simulink model "FCS_MPC_6ph_Regelungsmodell"  (R2022a)
settings: Solver=ode23t  StartTime=0.0  StopTime=0.1  RelTol=1e-3  AbsTol=1e-3  EnableMultiTasking=on
values from neighbouring files (symbols this model uses):
  f_c = 100000    [Params_testbench.m]
  L_d = 0.0001473    [Params_testbench.m]
  L_q = 0.0001484    [Params_testbench.m]
  L_x = 0.00005566    (= 5.566e-05)    [Params_testbench.m]
  L_y = L_x    (= 5.566e-05)    [Params_testbench.m]
  p = 5    [Params_testbench.m]
  psi_pm = 0.0048    [Params_testbench.m]
  R_ph = 0.1278    [Params_testbench.m]
  T_100MHz = 1/f_100MHz    (= 1e-08)    [Params_testbench.m]
  u_dc = 36.0    (= 36)    [Params_testbench.m]
libraries: hdlsllib x53, nesl_utility x39, fl_lib x32, ee_lib x12, simulink x8, spsAlphaBetaZerotodq0Lib x1
(part 2 of 8)

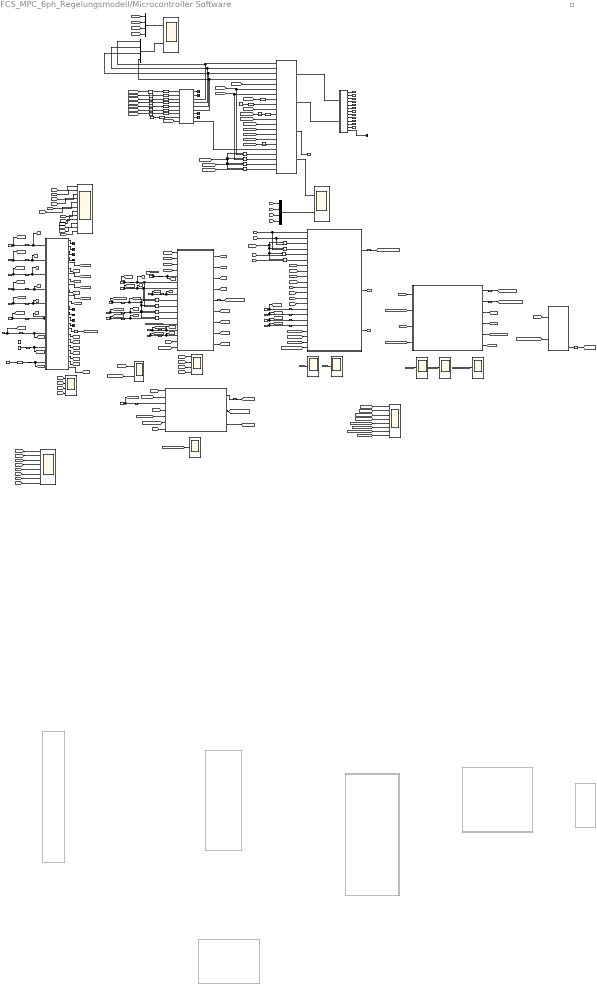
== system FCS_MPC_6ph_Regelungsmodell/Microcontroller Software ==
  note: IP-Core FCS_MPC_6Phase_PMSM
  note: IP-Core FCS_MPC_switching_states_2_level_inverter
  note: IP-Core VSD_and_Park_transformation
  i_a1 : Inport
  i_b1 : Inport  Port=2
  i_c1 : Inport  Port=3
  i_a2 : Inport  Port=4
  i_b2 : Inport  Port=5
  i_c2 : Inport  Port=6
  omega_m : Inport  Port=7
  theta_el : Inport  Port=8
  Rs : Inport  Port=9
  Ld : Inport  Port=10
  Lq : Inport  Port=11
  Lx : Inport  Port=12
  Ly : Inport  Port=13
  psiPM : Inport  Port=14
  SampleTime : Inport  Port=15
  id_ref : Inport  Port=16
  iq_ref : Inport  Port=17
  ix_ref : Inport  Port=18
  iy_ref : Inport  Port=19
  u_dc_link : Inport  Port=20
  pole_pairs : Inport  Port=21
  Ablauf : Scope  NumInputPorts=8
  Constant : Constant  Value=0
  Constant1 : Constant  Value=0  OutDataTypeStr=single  SampleTime=-1
  Constant2 : Constant  Value=0  OutDataTypeStr=fixdt(1,24,20)  SampleTime=-1
  Constant3 : Constant  Value=0
  Data Type Conversion{1..2,11..12} (4 alike) : DataTypeConversion  OutDataTypeStr=fixdt(1,24,20)  SaturateOnIntegerOverflow=off  RndMeth=Floor
  Data Type Conversion{5..10} (6 alike) : DataTypeConversion  OutDataTypeStr=fixdt(1,18,11)  SaturateOnIntegerOverflow=off  RndMeth=Floor
  Data Type Conversion13 : DataTypeConversion  OutDataTypeStr=fixdt(1,24,11)  SaturateOnIntegerOverflow=off  RndMeth=Floor
  Data Type Conversion4 : DataTypeConversion  OutDataTypeStr=boolean  RndMeth=Simplest  SaturateOnIntegerOverflow=off
  Delay1 : Delay  DelayLength=36
  Delay2 : Delay  DelayLength=21
  Delay22 : Delay  DelayLength=3
  Delay3 : Delay  DelayLength=66
  Delay4 : Delay  DelayLength=5
  Delay5 : Delay  DelayLength=5
  Delay6 : Delay
  Delay_compensation : Subsystem  TreatAsAtomicUnit=on
  Delay_compensation1 : Subsystem  Commented=on  TreatAsAtomicUnit=on
  Delay_compensation_phase_currents : Scope  NumInputPorts=4
  Divide{,1..11} (12 alike) : Product  Inputs=*/  RndMeth=Zero  SaturateOnIntegerOverflow=on
  Index : Scope
  J : Scope
  Min_cost_function_and_vopt1 : Subsystem  Commented=on  TreatAsAtomicUnit=on
  Min_cost_function_and_vopt2 : Subsystem  TreatAsAtomicUnit=on
  Mux : Mux
  Mux1 : Mux
  Mux2 : Mux
  Phase_voltages_per_switching_state1 : Subsystem  Commented=on  TreatAsAtomicUnit=on
  Phase_voltages_per_switching_state2 : Subsystem  TreatAsAtomicUnit=on
  Phase_voltages_per_switching_states : Scope
  Prediction_and_cost_function : Subsystem  TreatAsAtomicUnit=on
  Prediction_and_cost_function1 : Subsystem  Commented=on  TreatAsAtomicUnit=on
  Pulse Generator3 : DiscretePulseGenerator  PulseType=Time based  Period=1/100000  PulseWidth=0.1
  Pulse Generator4 : DiscretePulseGenerator  Commented=on  PulseType=Time based  Period=1/100000  PulseWidth=5
  Rate Transition{1..23} (23 alike) : RateTransition  OutPortSampleTime=1.0000e-08
  Subsystem2 : Subsystem
  Subsystem3 : Subsystem
  Subsystem5 : Subsystem  TreatAsAtomicUnit=on
  Switching_states : Subsystem  TreatAsAtomicUnit=on
  Switching_states1 : Subsystem  Commented=on  TreatAsAtomicUnit=on
  Terminator{,1..12} (13 alike) : Terminator
  Unit Delay{1..9} (9 alike) : UnitDelay  SampleTime=1/f_c  HasFrameUpgradeWarning=on
  VSD_and_Park_transformed_phase_currents : Scope  NumInputPorts=4
  last_applied_optimal_voltages : Scope
  min_Index_AXI : Scope
  min_J_AXI : Scope
  phase_currents : Scope  NumInputPorts=8
  phase_currents1 : Scope  NumInputPorts=12
  phase_currents2 : Scope  NumInputPorts=2
  phase_currents3 : Scope  NumInputPorts=2
  theta_test : Scope  NumInputPorts=2
  vsd_and_park_tra : Subsystem  TreatAsAtomicUnit=on
  vsd_and_park_tra1 : Subsystem  Commented=on  TreatAsAtomicUnit=on
  HB1T1 : Outport
  HB1B1 : Outport  Port=2
  HB2T1 : Outport  Port=3
  HB2B1 : Outport  Port=4
  HB3T1 : Outport  Port=5
  HB3B1 : Outport  Port=6
  HB4T : Outport  Port=7
  HB4B : Outport  Port=8
  HB5T : Outport  Port=9
  HB5B : Outport  Port=10
  HB6T : Outport  Port=11
  HB6B : Outport  Port=12
  v_opt : Outport  Port=13
  wires:
  Pulse Generator3/1 -> Data Type Conversion4/1
  vsd_and_park_tra/17(done) -> Delay22/1
  vsd_and_park_tra/4(i_beta_axi) -> Terminator1/1
  vsd_and_park_tra/10(i_x_axi) -> [i_x_AXI]
  vsd_and_park_tra/16(i_0_minus_axi) -> Terminator7/1
  Constant1/1 -> Rate Transition7/1  "i_a1_IP_Core"
  vsd_and_park_tra/12(i_y_axi) -> [i_y_AXI]
  vsd_and_park_tra/14(i_0_plus_axi) -> Terminator6/1
  vsd_and_park_tra/8(i_q_axi) -> [i_q_AXI]
  vsd_and_park_tra/6(i_d_axi) -> [i_d_AXI]
  vsd_and_park_tra/2(i_alpha_axi) -> Terminator/1
  i_a1/1 -> Rate Transition23/1, [i_a1_without_RT]  "i_a1_IP_Core"
  i_c2/1 -> Rate Transition5/1, [i_c2_without_RT]  "i_c2_IP_Core"
  i_b2/1 -> Rate Transition4/1, [i_b2_without_RT]  "i_b2_IP_Core"
  i_a2/1 -> Rate Transition3/1, [i_a2_without_RT]  "i_a2_IP_Core"
  i_c1/1 -> Rate Transition2/1, [i_c1_without_RT]  "i_c1_IP_Core"
  i_b1/1 -> Rate Transition1/1, [i_b1_without_RT]  "i_b1_IP_Core"
  vsd_and_park_tra/1(i_alpha) -> Terminator9/1  "i_alpha"
  vsd_and_park_tra/3(i_beta) -> Terminator10/1  "i_beta"
  vsd_and_park_tra/13(i_0_plus) -> Terminator11/1  "i_0_plus"
  vsd_and_park_tra/15(i_0_minus) -> Terminator12/1  "i_0_minus"
  vsd_and_park_tra/18(i_a1_axi) -> [i_a1_AXI]
  vsd_and_park_tra/19(i_b1_axi) -> [i_b1_AXI]
  vsd_and_park_tra/20(i_c1_axi) -> [i_c1_AXI]
  vsd_and_park_tra/21(i_a2_axi) -> [i_a2_AXI]
  vsd_and_park_tra/22(i_b2_axi) -> [i_b2_AXI]
  vsd_and_park_tra/23(i_c2_axi) -> [i_c2_AXI]
  [i_a1_AXI] -> phase_currents1/1
  [i_b1_AXI] -> phase_currents1/2
  [i_c1_AXI] -> phase_currents1/3
  [i_a2_AXI] -> phase_currents1/4
  [i_b2_AXI] -> phase_currents1/5
  [i_c2_AXI] -> phase_currents1/6
  [i_d_AXI] -> VSD_and_Park_transformed_phase_currents/1
  [i_q_AXI] -> VSD_and_Park_transformed_phase_currents/2
  [i_y_AXI] -> VSD_and_Park_transformed_phase_currents/4
  [i_x_AXI] -> VSD_and_Park_transformed_phase_currents/3
  Divide1/1 -> Delay_compensation/10(SampleTime_div_Lq_AXI)
  Divide/1 -> Delay_compensation/9(SampleTime_div_Ld_AXI)
  Delay_compensation/2(iq_k_1) -> [iq_k_1]
  Divide2/1 -> Delay_compensation/11(SampleTime_div_Lx_AXI)
  Delay_compensation/1(id_k_1) -> [id_k_1]
  Delay_compensation/4(iy_k_1) -> [iy_k_1]
  Delay_compensation/3(ix_k_1) -> [ix_k_1]
  Divide3/1 -> Delay_compensation/12(SampleTime_div_Ly_AXI)
  psiPM/1 -> Rate Transition9/1, [psiPM_without_RT]  "i_d"
  Lq/1 -> Rate Transition10/1, [Lq_without_RT]  "i_a1_IP_Core"
  Ld/1 -> Rate Transition11/1, [Ld_without_RT]  "i_a1_IP_Core"
  Rs/1 -> Rate Transition12/1, [Rs_without_RT]  "i_a1_IP_Core"
  Lx/1 -> Rate Transition14/1, [Lx_without_RT]  "i_a1_IP_Core"
  Ly/1 -> Rate Transition15/1, [Ly_without_RT]  "i_a1_IP_Core"
  pole_pairs/1 -> Rate Transition16/1, [pole_pairs_without_RT]  "i_a1_IP_Core"
  omega_m/1 -> Rate Transition17/1, [omega_m_without_RT]  "i_d"
  [valid_in_ADC] -> Delay_compensation/16(valid_in_ADC)
  [done_VSD_and_Park] -> Delay_compensation/17(valid_in)
  vsd_and_park_tra/5(i_d) -> [i_d_measured]  "i_d"
  vsd_and_park_tra/7(i_q) -> [i_q_measured]  "i_q"
  vsd_and_park_tra/9(i_x) -> [i_x_measured]  "i_x"
  vsd_and_park_tra/11(i_y) -> [i_y_measured]  "i_y"
  [i_d_measured] -> Delay_compensation/1(id_measured)
  [i_q_measured] -> Delay_compensation/2(iq_measured)
  [i_x_measured] -> Delay_compensation/3(ix_measured)
  [i_y_measured] -> Delay_compensation/4(iy_measured)
  Delay_compensation/6(id_k_1_AXI) -> [id_k_1_AXI]
  Delay_compensation/7(iq_k_1_AXI) -> [iq_k_1_AXI]
  Delay_compensation/8(ix_k_1_AXI) -> [ix_k_1_AXI]
  Delay_compensation/9(iy_k_1_AXI) -> [iy_k_1_AXI]
  [id_k_1_AXI] -> Delay_compensation_phase_currents/1
  [iq_k_1_AXI] -> Delay_compensation_phase_currents/2
  [ix_k_1_AXI] -> Delay_compensation_phase_currents/3
  [iy_k_1_AXI] -> Delay_compensation_phase_currents/4
  [theta_el] -> Phase_voltages_per_switching_state2/1(theta_el)
  [theta_el_offset_AXI] -> Phase_voltages_per_switching_state2/2(theta_el_offset_AXI)
  u_dc_link/1 -> Rate Transition22/1, [u_dc_link_without_RT]  "i_a1_IP_Core"
  Delay_compensation/5(done) -> Delay1/1
  [valid_in_delay_compensation] -> Phase_voltages_per_switching_state2/5(valid_in_delay_compensation)
  [valid_in_ADC] -> Phase_voltages_per_switching_state2/7(valid_in_ADC)
  Phase_voltages_per_switching_state2/1(done) -> Delay2/1
  Phase_voltages_per_switching_state2/2(phase_voltages_per_switching_state) -> [phase_voltages_per_switching_states]
  [phase_voltages_per_switching_states] -> Phase_voltages_per_switching_states/1
  Divide6/1 -> Prediction_and_cost_function/5(SampleTime_div_Lx_AXI)
  [psiPM] -> Prediction_and_cost_function/14(psiPM_AXI)
  Divide7/1 -> Prediction_and_cost_function/6(SampleTime_div_Ly_AXI)
  [Ld] -> Divide4/2, Prediction_and_cost_function/2(Ld_AXI)
  [omega_m] -> Prediction_and_cost_function/12(omega_m_measured)
  [SampleTime] -> Divide5/1, Divide7/1, Divide6/1, Divide4/1
  [Lq] -> Divide5/2, Prediction_and_cost_function/1(Lq_AXI)
  Divide4/1 -> Prediction_and_cost_function/3(SampleTime_div_Ld_AXI)
  [Rs] -> Prediction_and_cost_function/11(Rs_AXI)
  [Ly] -> Divide7/2
  [Lx] -> Divide6/2
  Prediction_and_cost_function/2(Index) -> [Index]
  Divide5/1 -> Prediction_and_cost_function/4(SampleTime_div_Lq_AXI)
  [pole_pairs] -> Prediction_and_cost_function/13(pole_pairs_AXI)
  Prediction_and_cost_function/3(J) -> [J]
  [J] -> J/1
  [Index] -> Index/1
  Prediction_and_cost_function/1(done) -> Delay3/1
  [id_k_1] -> Prediction_and_cost_function/7(id_k_1)
  [iq_k_1] -> Prediction_and_cost_function/8(iq_k_1)
  [ix_k_1] -> Prediction_and_cost_function/9(ix_k_1)
  [iy_k_1] -> Prediction_and_cost_function/10(iy_k_1)
  id_ref/1 -> Rate Transition18/1, [id_ref_without_RT]  "i_a1_IP_Core"
  iq_ref/1 -> Rate Transition19/1, [iq_ref_without_RT]  "i_a1_IP_Core"
  ix_ref/1 -> Rate Transition20/1, [ix_ref_without_RT]  "i_a1_IP_Core"
  iy_ref/1 -> Rate Transition21/1, [iy_ref_without_RT]  "i_a1_IP_Core"
  [valid_in_phase_voltages] -> Prediction_and_cost_function/19(valid_in)
  [done_VSD_and_Park] -> Prediction_and_cost_function/20(Reset)
  [valid_in_ADC] -> Prediction_and_cost_function/21(valid_in_ADC)
  [phase_voltages_per_switching_states] -> Prediction_and_cost_function/22(dqxy_phase_voltage_per_switching_state)
  Min_cost_function_and_vopt2/6(Index_AXI) -> [min_Index_AXI]
  Min_cost_function_and_vopt2/2(done_complete) -> Delay5/1
  Min_cost_function_and_vopt2/3(J_AXI) -> [min_J_AXI]
  Min_cost_function_and_vopt2/1(done) -> Delay4/1
  Min_cost_function_and_vopt2/4(Index) -> [min_Index]
  Min_cost_function_and_vopt2/5(voltages) -> [last_applied_optimal_voltages]
  [Index] -> Min_cost_function_and_vopt2/1(Index_in)
  [Index] -> Phase_voltages_per_switching_state2/4(Index)
  [valid_in_prediction_and_cost_function] -> Min_cost_function_and_vopt2/2(valid_in)
  [J] -> Min_cost_function_and_vopt2/3(J_in)
  [phase_voltages_per_switching_states] -> Min_cost_function_and_vopt2/4(phase_voltages_per_switching_state_in)
  [min_J_AXI] -> min_J_AXI/1
  [min_Index_AXI] -> min_Index_AXI/1
  [last_applied_optimal_voltages] -> last_applied_optimal_voltages/1
  [last_applied_optimal_voltages] -> Delay_compensation/13(last_applied_optimal_voltages_in)
  [valid_in_done_min_cost_function] -> Phase_voltages_per_switching_state2/6(valid_in_min_cost_function-and_vopt)
  Switching_states/13(done) -> Delay6/1
  [min_Index] -> Switching_states/1(I)
  [valid_in_done_complete_min_cost_function] -> Switching_states/2(valid_in)
  [valid_in_ADC] -> Ablauf/1  "valid_in_ADC"
  [done_VSD_and_Park] -> Ablauf/2  "done_VSD_and_Park"
  [valid_in_delay_compensation] -> Ablauf/3  "done_delay_compensation"
  [valid_in_phase_voltages] -> Ablauf/4  "done_phase_voltages"
  [valid_in_prediction_and_cost_function] -> Ablauf/5  "done_prediction_and_cost_function"
  [valid_in_done_min_cost_function] -> Ablauf/6  "done_min_cost_function"
  [valid_in_done_complete_min_cost_function] -> Ablauf/7  "done_complete_min_cost_function"
  [done_switching_states] -> Ablauf/8  "done_switching_states"
  Delay22/1 -> [done_VSD_and_Park]
  Delay1/1 -> [valid_in_delay_compensation]
  Delay2/1 -> [valid_in_phase_voltages]
  Delay3/1 -> [valid_in_prediction_and_cost_function]
  Delay4/1 -> [valid_in_done_min_cost_function]
  Delay5/1 -> [valid_in_done_complete_min_cost_function]
  Delay6/1 -> [done_switching_states]
  [id_k_1_AXI] -> phase_currents/1  "id_k_1"
  [iq_k_1_AXI] -> phase_currents/2  "iq_k_1"
  [ix_k_1_AXI] -> phase_currents/3  "ix_k_1"
  [iy_k_1_AXI] -> phase_currents/4  "iy_k_1"
  [i_d_AXI] -> phase_currents/5  "id"
  [i_q_AXI] -> phase_currents/6  "iq"
  [i_x_AXI] -> phase_currents/7  "ix"
  [i_y_AXI] -> phase_currents/8  "iy"
  Data Type Conversion4/1 -> Rate Transition8/1  "i_a1_IP_Core"
  SampleTime/1 -> Rate Transition13/1, [SampleTime_without_RT]  "i_a1_IP_Core"
  [i_a1] -> phase_currents1/7
  [i_b1] -> phase_currents1/8
  [i_c1] -> phase_currents1/9
  [i_a2] -> phase_currents1/10
  [i_b2] -> phase_currents1/11
  [i_c2] -> phase_currents1/12
  vsd_and_park_tra/24(theta_test) -> [theta_test_vsd]
  [theta_test_vsd] -> theta_test/1  "VSD"
  Phase_voltages_per_switching_state2/3(theta_test) -> [theta_test_phase_voltages]
  [theta_test_phase_voltages] -> theta_test/2  "phase_voltages"
  theta_el/1 -> Rate Transition6/1, [theta_el_without_RT]  "i_a1_IP_Core"
  Constant/1 -> Data Type Conversion1/1
  Divide11/1 -> Subsystem3/22(SampleTime_div_Ly_AXI)  "i_d"
  Subsystem2/1(i_alpha) -> Terminator4/1  "i_alpha"
  Subsystem3/1(I) -> Subsystem5/1(I)
  [Ld_without_RT] -> Subsystem3/6(Ld_AXI), Divide8/2  "i_d"
  Divide8/1 -> Subsystem3/19(SampleTime_div_Ld_AXI)  "i_d"
  Subsystem2/6(i_y) -> Subsystem3/4(i_y), Mux1/4  "i_y"
  Data Type Conversion2/1 -> Subsystem3/9(theta_el_offset_AXI)  "curent_valid_in"
  Divide10/1 -> Subsystem3/21(SampleTime_div_Lx_AXI)  "i_d"
  Constant3/1 -> Data Type Conversion2/1
  Subsystem2/5(i_x) -> Subsystem3/3(i_x), Mux1/3  "i_x"
  Subsystem3/3(v_opt) -> v_opt/1
  [Rs_without_RT] -> Subsystem3/5(Rs_AXI)  "i_d"
  Subsystem5/13(done) -> Terminator8/1  "done_switching_states"
  [Lq_without_RT] -> Divide9/2, Subsystem3/7(Lq_AXI)  "i_d"
  Subsystem2/4(i_q) -> Mux1/2, Subsystem3/2(i_q)  "i_q"
  Subsystem3/2(done) -> Subsystem5/2(valid_in)  "done_MPC"
  Subsystem2/3(i_d) -> Mux1/1, Subsystem3/1(i_d)  "i_d"
  Subsystem2/9(done) -> Subsystem3/18(valid_in)  "done_trans"
  [Ly_without_RT] -> Divide11/2
  [SampleTime_without_RT] -> Divide8/1, Divide9/1, Divide11/1, Divide10/1
  Divide9/1 -> Subsystem3/20(SampleTime_div_Lq_AXI)  "i_d"
  Subsystem2/2(i_beta) -> Terminator5/1  "i_beta"
  [Lx_without_RT] -> Divide10/2
  Subsystem2/8(i_0_minus) -> Terminator3/1  "i_0_minus"
  Data Type Conversion1/1 -> Subsystem2/8(theta_el_offset_AXI)  "curent_valid_in"
  Subsystem2/7(i_0_plus) -> Terminator2/1  "i_0_plus"
  Data Type Conversion5/1 -> Subsystem2/1(i_a1)  "curent_valid_in"
  Data Type Conversion6/1 -> Subsystem2/2(i_b1)  "curent_valid_in"
  Data Type Conversion7/1 -> Subsystem2/3(i_c1)  "curent_valid_in"
  Data Type Conversion8/1 -> Subsystem2/4(i_a2)  "curent_valid_in"
  Data Type Conversion9/1 -> Subsystem2/5(i_b2)  "curent_valid_in"
  Data Type Conversion10/1 -> Subsystem2/6(i_c2)  "curent_valid_in"
  [theta_el_without_RT] -> Unit Delay7/1  "curent_valid_in"
  [theta_el_without_RT] -> Data Type Conversion12/1
  Data Type Conversion11/1 -> Subsystem2/7(theta_el)  "curent_valid_in"
  Data Type Conversion12/1 -> Subsystem3/8(theta_el)  "curent_valid_in"
  [psiPM_without_RT] -> Subsystem3/10(psiPM_AXI)
  [pole_pairs_without_RT] -> Subsystem3/12(pole_pairs_AXI)
  [id_ref_without_RT] -> Subsystem3/13(id_ref_AXI)
  [iq_ref_without_RT] -> Subsystem3/14(iq_ref_AXI)
  [ix_ref_without_RT] -> Subsystem3/15(ix_ref_AXI)
  [iy_ref_without_RT] -> Subsystem3/16(iy_ref_AXI)
  Data Type Conversion13/1 -> Subsystem3/11(omega_m)
  [valid_in_ADC] -> Subsystem2/9(curent_valid_in)  "curent_valid_in"
  Mux/1 -> phase_currents2/1
  [i_d_measured] -> Mux/1
  [i_q_measured] -> Mux/2
  [i_x_measured] -> Mux/3
  [i_y_measured] -> Mux/4
  Mux1/1 -> phase_currents2/2
  [i_a1_without_RT] -> Unit Delay2/1
  [i_b1_without_RT] -> Unit Delay1/1
  [i_c1_without_RT] -> Unit Delay3/1
  [i_a2_without_RT] -> Unit Delay4/1
  [i_b2_without_RT] -> Unit Delay5/1
  [i_c2_without_RT] -> Unit Delay6/1
  [omega_m_without_RT] -> Unit Delay8/1
  [u_dc_link_without_RT] -> Unit Delay9/1
  Rate Transition23/1 -> [i_a1], vsd_and_park_tra/1(i_a1)  "i_a1_IP_Core"
  Rate Transition1/1 -> [i_b1], vsd_and_park_tra/2(i_b1)  "i_a1_IP_Core"
  Rate Transition2/1 -> [i_c1], vsd_and_park_tra/3(i_c1)  "i_a1_IP_Core"
  Rate Transition3/1 -> [i_a2], vsd_and_park_tra/4(i_a2)  "i_a1_IP_Core"
  Rate Transition4/1 -> [i_b2], vsd_and_park_tra/5(i_b2)  "i_a1_IP_Core"
  Rate Transition5/1 -> [i_c2], vsd_and_park_tra/6(i_c2)  "i_a1_IP_Core"
  Rate Transition6/1 -> [theta_el], vsd_and_park_tra/7(theta_el)  "i_a1_IP_Core"
  Rate Transition7/1 -> vsd_and_park_tra/8(theta_el_offset_), [theta_el_offset_AXI]  "i_a1_IP_Core"
  Rate Transition8/1 -> [valid_in_ADC], vsd_and_park_tra/9(curent_valid_in)  "i_a1_IP_Core"
  Rate Transition9/1 -> [psiPM], Delay_compensation/5(psiPM_AXI)  "i_a1_IP_Core"
  Rate Transition10/1 -> [Lq], Delay_compensation/6(Lq_AXI), Divide1/2  "i_a1_IP_Core"
  Rate Transition11/1 -> [Ld], Delay_compensation/7(Ld_AXI), Divide/2  "i_a1_IP_Core"
  Rate Transition12/1 -> [Rs], Delay_compensation/8(Rs_AXI)  "i_a1_IP_Core"
  Rate Transition13/1 -> Divide/1, Divide1/1, Divide3/1, Divide2/1, [SampleTime]  "i_a1_IP_Core"
  Rate Transition14/1 -> [Lx], Divide2/2  "i_a1_IP_Core"
  Rate Transition15/1 -> [Ly], Divide3/2  "i_a1_IP_Core"
  Rate Transition16/1 -> [pole_pairs], Delay_compensation/14(pole_pairs_AXI)  "i_a1_IP_Core"
  Rate Transition17/1 -> [omega_m], Delay_compensation/15(omega_m_measured)  "i_a1_IP_Core"
  Rate Transition18/1 -> Prediction_and_cost_function/15(id_ref_AXI)  "i_a1_IP_Core"
  Rate Transition19/1 -> Prediction_and_cost_function/16(iq_ref_AXI)  "i_a1_IP_Core"
  Rate Transition20/1 -> Prediction_and_cost_function/17(ix_ref_AXI)  "i_a1_IP_Core"
  Rate Transition21/1 -> Prediction_and_cost_function/18(iy_ref_AXI)  "i_a1_IP_Core"
  Rate Transition22/1 -> Phase_voltages_per_switching_state2/3(u_dc_link_voltage_AXI)  "i_a1_IP_Core"
  Unit Delay2/1 -> Data Type Conversion5/1
  Unit Delay1/1 -> Data Type Conversion6/1
  Unit Delay3/1 -> Data Type Conversion7/1
  Unit Delay4/1 -> Data Type Conversion8/1
  Unit Delay5/1 -> Data Type Conversion9/1
  Unit Delay6/1 -> Data Type Conversion10/1
  Unit Delay7/1 -> Data Type Conversion11/1
  Unit Delay8/1 -> Data Type Conversion13/1
  Unit Delay9/1 -> Subsystem3/17(u_dc_link_AXI)
  Subsystem5/2(HB1B) -> HB1B1/1
  Subsystem5/1(HB1T) -> HB1T1/1
  Subsystem5/3(HB2T) -> HB2T1/1
  Subsystem5/4(HB2B) -> HB2B1/1
  Subsystem5/5(HB3T) -> HB3T1/1
  Subsystem5/6(HB3B) -> HB3B1/1
  Subsystem5/7(HB4T) -> HB4T/1
  Subsystem5/8(HB4B) -> HB4B/1
  Subsystem5/9(HB5T) -> HB5T/1
  Subsystem5/10(HB5B) -> HB5B/1
  Subsystem5/11(HB6T) -> HB6T/1
  Subsystem5/12(HB6B) -> HB6B/1
  Subsystem3/4(Prediction_old) -> phase_currents3/1
  [id_k_1] -> Mux2/1
  [iq_k_1] -> Mux2/2
  [ix_k_1] -> Mux2/3
  [iy_k_1] -> Mux2/4
  Mux2/1 -> phase_currents3/2

== system FCS_MPC_6ph_Regelungsmodell/Power_Source ==
  Controlled Voltage Source : fl_lib/Electrical/Electrical Sources/Controlled Voltage Source
      settings: SourceProductBaseCode=PW,SS,VE
  + : PMIOPort  Side=Right
  - : PMIOPort  Port=2  Side=Right
  ref_voltage : PMIOPort  Port=3  Side=Left
  connections:
  Controlled Voltage Source/LConn1 -- +/RConn1
  Controlled Voltage Source/RConn2 -- -/RConn1
  Controlled Voltage Source/RConn1 -- ref_voltage/RConn1

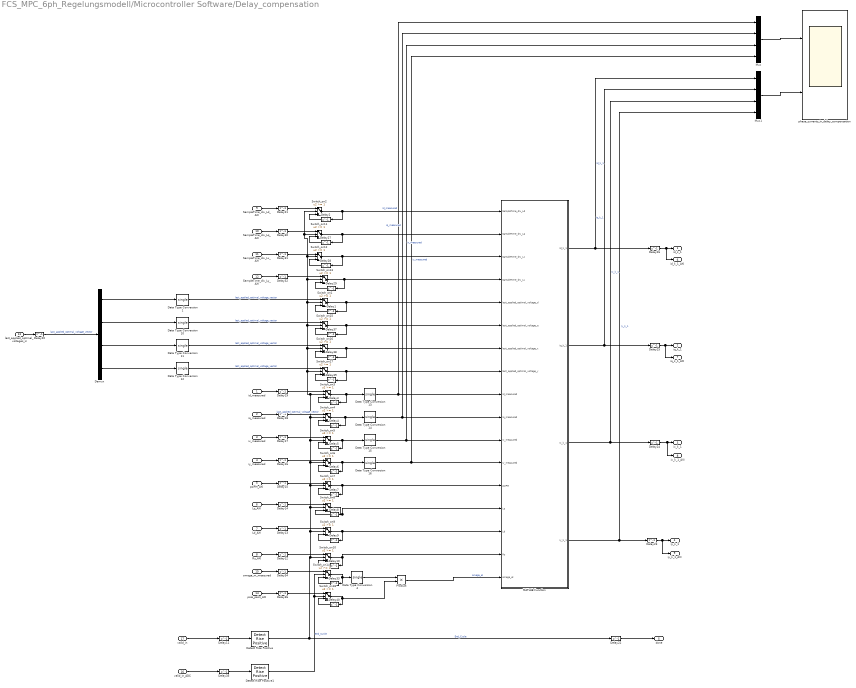
== system FCS_MPC_6ph_Regelungsmodell/Microcontroller Software/Delay_compensation ==
  id_measured : Inport
  iq_measured : Inport  Port=2
  ix_measured : Inport  Port=3
  iy_measured : Inport  Port=4
  psiPM_AXI : Inport  Port=5
  Lq_AXI : Inport  Port=6
  Ld_AXI : Inport  Port=7
  Rs_AXI : Inport  Port=8
  SampleTime_div_Ld_AXI : Inport  Port=9
  SampleTime_div_Lq_AXI : Inport  Port=10
  SampleTime_div_Lx_AXI : Inport  Port=11
  SampleTime_div_Ly_AXI : Inport  Port=12
  last_applied_optimal_voltages_in : Inport  Port=13
  pole_pairs_AXI : Inport  Port=14
  omega_m_measured : Inport  Port=15
  valid_in_ADC : Inport  Port=16
  valid_in : Inport  Port=17
  Data Type Conversion{1,4,10..16} (9 alike) : DataTypeConversion  OutDataTypeStr=single  RndMeth=Nearest  SaturateOnIntegerOverflow=off
  Delay{1..40} (40 alike) : Delay  DelayLength=1
  Demux : Demux
  Detect Rise Positive : hdlsllib/Logic and Bit Operations/Detect Rise Positive  vinit=0  OutDataTypeStr=boolean
      settings: SourceProductBaseCode=SL
  Detect Rise Positive1 : hdlsllib/Logic and Bit Operations/Detect Rise Positive  vinit=0  OutDataTypeStr=boolean
      settings: SourceProductBaseCode=SL
  MATLAB Function : MATLAB Function  TreatAsAtomicUnit=on
  Mux : Mux
  Mux1 : Mux
  Product : Product  Inputs=**
  Switch_on{1..13,15..18} (17 alike) : Switch  Threshold=1  OutDataTypeStr=single  RndMeth=Simplest  SaturateOnIntegerOverflow=off  InputSameDT=off
  Switch_on14 : Switch  Threshold=1  RndMeth=Simplest  SaturateOnIntegerOverflow=off  InputSameDT=off  OutDataTypeStr=Inherit: Same as first input
  phase_currents_in_delay_compensation : Scope  NumInputPorts=2
  id_k_1 : Outport
  iq_k_1 : Outport  Port=2
  ix_k_1 : Outport  Port=3
  iy_k_1 : Outport  Port=4
  done : Outport  Port=5
  id_k_1_AXI : Outport  Port=6
  iq_k_1_AXI : Outport  Port=7
  ix_k_1_AXI : Outport  Port=8
  iy_k_1_AXI : Outport  Port=9
  wires:
  Switch_on14/1 -> Data Type Conversion4/1, Delay33/1
  Delay33/1 -> Switch_on14/3
  pole_pairs_AXI/1 -> Delay36/1
  Delay9/1 -> Switch_on9/3
  Switch_on9/1 -> Delay9/1, MATLAB Function/15(Ld)
  Delay32/1 -> Switch_on13/1
  Lq_AXI/1 -> Delay14/1
  Delay31/1 -> Switch_on12/1
  Switch_on12/1 -> Delay28/1, MATLAB Function/3(SampleTime_div_Lx)
  Delay30/1 -> Switch_on11/1
  Delay29/1 -> Switch_on13/3
  SampleTime_div_Lx_AXI/1 -> Delay31/1
  Delay26/1 -> id_k_1_AXI/1, id_k_1/1
  Product/1 -> MATLAB Function/17(omega_el)  "omega_el"
  Delay11/1 -> Detect Rise Positive/1
  Delay2/1 -> Switch_on2/3
  SampleTime_div_Lq_AXI/1 -> Delay30/1
  Switch_on5/1 -> Delay5/1, Data Type Conversion15/1
  Delay12/1 -> Switch_on10/1
  Rs_AXI/1 -> Delay12/1
  Delay1/1 -> Switch_on1/3
  Delay27/1 -> Switch_on11/3
  Delay21/1 -> Switch_on2/1
  Delay23/1 -> iy_k_1_AXI/1, iy_k_1/1
  Delay24/1 -> ix_k_1_AXI/1, ix_k_1/1
  Delay20/1 -> Demux/1  "last_applied_optimal_voltage_vector"
  Switch_on1/1 -> Delay1/1, MATLAB Function/5(last_applied_optimal_voltage_d)
  Delay8/1 -> Switch_on8/3
  Delay10/1 -> Switch_on10/3
  valid_in/1 -> Delay11/1
  Switch_on6/1 -> Delay6/1, Data Type Conversion16/1
  psiPM_AXI/1 -> Delay15/1
  Delay25/1 -> iq_k_1_AXI/1, iq_k_1/1
  Switch_on13/1 -> Delay29/1, MATLAB Function/4(SampleTime_div_Ly)
  Switch_on4/1 -> Delay4/1, Data Type Conversion14/1
  Delay15/1 -> Switch_on7/1
  SampleTime_div_Ly_AXI/1 -> Delay32/1
  Switch_on10/1 -> Delay10/1, MATLAB Function/16(Rs)
  Delay7/1 -> Switch_on7/3
  Delay28/1 -> Switch_on12/3
  Switch_on8/1 -> Delay8/1, MATLAB Function/14(Lq)
  Ld_AXI/1 -> Delay13/1
  Delay6/1 -> Switch_on6/3
  Delay4/1 -> Switch_on4/3
  Switch_on11/1 -> Delay27/1, MATLAB Function/2(SampleTime_div_Lq)
  Delay3/1 -> Switch_on3/3
  Delay14/1 -> Switch_on8/1
  Switch_on2/1 -> Delay2/1, MATLAB Function/1(SampleTime_div_Ld)
  Delay22/1 -> done/1
  Switch_on3/1 -> Delay3/1, Data Type Conversion13/1
  Delay13/1 -> Switch_on9/1
  Delay5/1 -> Switch_on5/3
  SampleTime_div_Ld_AXI/1 -> Delay21/1
  last_applied_optimal_voltages_in/1 -> Delay20/1
  id_measured/1 -> Delay19/1
  iq_measured/1 -> Delay18/1
  ix_measured/1 -> Delay17/1
  iy_measured/1 -> Delay16/1
  omega_m_measured/1 -> Delay34/1
  Delay35/1 -> Detect Rise Positive1/1
  valid_in_ADC/1 -> Delay35/1
  Delay34/1 -> Switch_on14/1
  Delay36/1 -> Switch_on18/1
  Demux/1 -> Data Type Conversion1/1
  Delay37/1 -> Switch_on15/3
  Switch_on15/1 -> MATLAB Function/6(last_applied_optimal_voltage_q), Delay37/1
  Demux/2 -> Data Type Conversion10/1
  Delay38/1 -> Switch_on16/3
  Switch_on16/1 -> MATLAB Function/7(last_applied_optimal_voltage_x), Delay38/1
  Demux/3 -> Data Type Conversion11/1
  Delay39/1 -> Switch_on17/3
  Detect Rise Positive/1 -> Switch_on17/2, Switch_on16/2, Switch_on15/2, Switch_on13/2, Switch_on2/2, Switch_on11/2, Switch_on12/2, Switch_on1/2, Switch_on3/2, Switch_on4/2, Switch_on5/2, Switch_on6/2, Switch_on7/2, Switch_on8/2, Switch_on9/2, Switch_on10/2, Delay22/1  "End_Cycle"
  Switch_on17/1 -> MATLAB Function/8(last_applied_optimal_voltage_y), Delay39/1
  Demux/4 -> Data Type Conversion12/1
  Data Type Conversion1/1 -> Switch_on1/1  "last_applied_optimal_voltage_vector"
  Data Type Conversion10/1 -> Switch_on15/1  "last_applied_optimal_voltage_vector"
  Data Type Conversion11/1 -> Switch_on16/1  "last_applied_optimal_voltage_vector"
  Data Type Conversion12/1 -> Switch_on17/1  "last_applied_optimal_voltage_vector"
  Delay19/1 -> Switch_on3/1
  Delay18/1 -> Switch_on4/1  "last_applied_optimal_voltage_vector"
  Delay17/1 -> Switch_on5/1
  Delay16/1 -> Switch_on6/1
  Data Type Conversion4/1 -> Product/1
  MATLAB Function/1(id_k_1) -> Mux1/1, Delay26/1  "id_k_1"
  MATLAB Function/2(iq_k_1) -> Mux1/2, Delay25/1  "iq_k_1"
  MATLAB Function/3(ix_k_1) -> Mux1/3, Delay24/1  "ix_k_1"
  MATLAB Function/4(iy_k_1) -> Mux1/4, Delay23/1  "iy_k_1"
  Switch_on18/1 -> Product/2, Delay40/1
  Detect Rise Positive1/1 -> Switch_on18/2, Switch_on14/2  "End_Cycle"
  Delay40/1 -> Switch_on18/3
  Data Type Conversion13/1 -> Mux/1, MATLAB Function/9(id_measured)  "id_measured"
  Data Type Conversion14/1 -> Mux/2, MATLAB Function/10(iq_measured)  "iq_measured"
  Data Type Conversion15/1 -> Mux/3, MATLAB Function/11(ix_measured)  "ix_measured"
  Data Type Conversion16/1 -> Mux/4, MATLAB Function/12(iy_measured)  "iy_measured"
  Switch_on7/1 -> MATLAB Function/13(psiPM), Delay7/1
  Mux/1 -> phase_currents_in_delay_compensation/1
  Mux1/1 -> phase_currents_in_delay_compensation/2

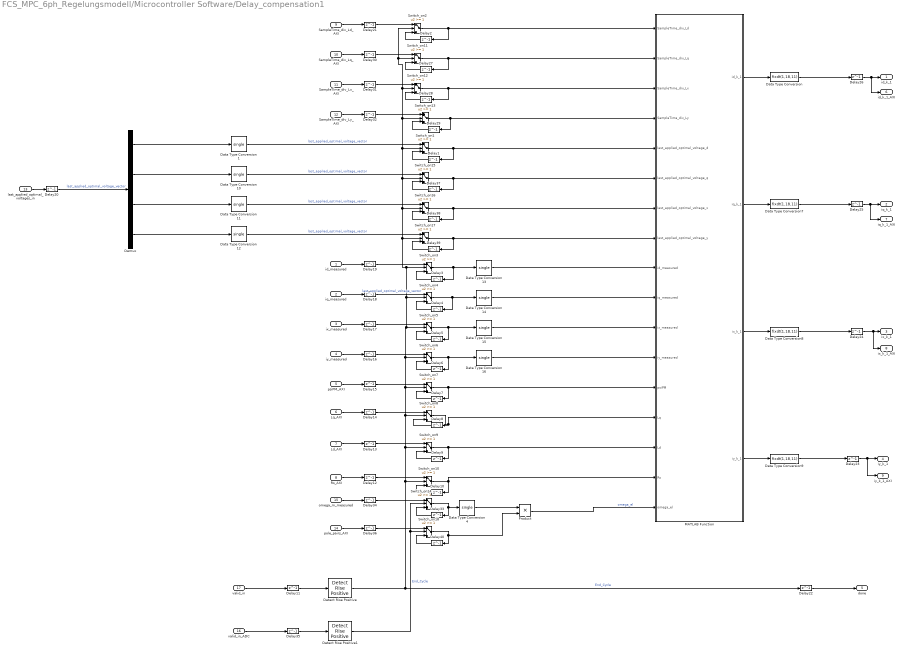
== system FCS_MPC_6ph_Regelungsmodell/Microcontroller Software/Delay_compensation1 ==
  id_measured : Inport
  iq_measured : Inport  Port=2
  ix_measured : Inport  Port=3
  iy_measured : Inport  Port=4
  psiPM_AXI : Inport  Port=5
  Lq_AXI : Inport  Port=6
  Ld_AXI : Inport  Port=7
  Rs_AXI : Inport  Port=8
  SampleTime_div_Ld_AXI : Inport  Port=9
  SampleTime_div_Lq_AXI : Inport  Port=10
  SampleTime_div_Lx_AXI : Inport  Port=11
  SampleTime_div_Ly_AXI : Inport  Port=12
  last_applied_optimal_voltages_in : Inport  Port=13
  pole_pairs_AXI : Inport  Port=14
  omega_m_measured : Inport  Port=15
  valid_in_ADC : Inport  Port=16
  valid_in : Inport  Port=17
  Data Type Conversion{,7..9} (4 alike) : DataTypeConversion  OutDataTypeStr=fixdt(1,18,11)  SaturateOnIntegerOverflow=off  RndMeth=Floor
  Data Type Conversion{1,4,10..16} (9 alike) : DataTypeConversion  OutDataTypeStr=single  RndMeth=Nearest  SaturateOnIntegerOverflow=off
  Delay{1..40} (40 alike) : Delay  DelayLength=1
  Demux : Demux
  Detect Rise Positive : hdlsllib/Logic and Bit Operations/Detect Rise Positive  vinit=0  OutDataTypeStr=boolean
      settings: SourceProductBaseCode=SL
  Detect Rise Positive1 : hdlsllib/Logic and Bit Operations/Detect Rise Positive  vinit=0  OutDataTypeStr=boolean
      settings: SourceProductBaseCode=SL
  MATLAB Function : MATLAB Function  TreatAsAtomicUnit=on
  Product : Product  Inputs=**
  Switch_on{1..13,15..18} (17 alike) : Switch  Threshold=1  OutDataTypeStr=single  RndMeth=Simplest  SaturateOnIntegerOverflow=off  InputSameDT=off
  Switch_on14 : Switch  Threshold=1  RndMeth=Simplest  SaturateOnIntegerOverflow=off  InputSameDT=off  OutDataTypeStr=Inherit: Same as first input
  id_k_1 : Outport
  iq_k_1 : Outport  Port=2
  ix_k_1 : Outport  Port=3
  iy_k_1 : Outport  Port=4
  done : Outport  Port=5
  id_k_1_AXI : Outport  Port=6
  iq_k_1_AXI : Outport  Port=7
  ix_k_1_AXI : Outport  Port=8
  iy_k_1_AXI : Outport  Port=9
  wires:
  Switch_on14/1 -> Data Type Conversion4/1, Delay33/1
  Delay33/1 -> Switch_on14/3
  pole_pairs_AXI/1 -> Delay36/1
  Delay9/1 -> Switch_on9/3
  Switch_on9/1 -> Delay9/1, MATLAB Function/15(Ld)
  Delay32/1 -> Switch_on13/1
  MATLAB Function/2(iq_k_1) -> Data Type Conversion7/1
  Lq_AXI/1 -> Delay14/1
  Delay31/1 -> Switch_on12/1
  Switch_on12/1 -> Delay28/1, MATLAB Function/3(SampleTime_div_Lx)
  Delay30/1 -> Switch_on11/1
  Delay29/1 -> Switch_on13/3
  SampleTime_div_Lx_AXI/1 -> Delay31/1
  Delay26/1 -> id_k_1_AXI/1, id_k_1/1
  Product/1 -> MATLAB Function/17(omega_el)  "omega_el"
  Delay11/1 -> Detect Rise Positive/1
  Delay2/1 -> Switch_on2/3
  SampleTime_div_Lq_AXI/1 -> Delay30/1
  Switch_on5/1 -> Delay5/1, Data Type Conversion15/1
  Delay12/1 -> Switch_on10/1
  Rs_AXI/1 -> Delay12/1
  Delay1/1 -> Switch_on1/3
  MATLAB Function/3(ix_k_1) -> Data Type Conversion8/1
  Delay27/1 -> Switch_on11/3
  Delay21/1 -> Switch_on2/1
  Delay23/1 -> iy_k_1_AXI/1, iy_k_1/1
  MATLAB Function/1(id_k_1) -> Data Type Conversion/1
  Delay24/1 -> ix_k_1_AXI/1, ix_k_1/1
  Delay20/1 -> Demux/1  "last_applied_optimal_voltage_vector"
  Switch_on1/1 -> Delay1/1, MATLAB Function/5(last_applied_optimal_voltage_d)
  Delay8/1 -> Switch_on8/3
  Delay10/1 -> Switch_on10/3
  valid_in/1 -> Delay11/1
  Switch_on6/1 -> Delay6/1, Data Type Conversion16/1
  MATLAB Function/4(iy_k_1) -> Data Type Conversion9/1
  psiPM_AXI/1 -> Delay15/1
  Delay25/1 -> iq_k_1_AXI/1, iq_k_1/1
  Switch_on13/1 -> Delay29/1, MATLAB Function/4(SampleTime_div_Ly)
  Switch_on4/1 -> Delay4/1, Data Type Conversion14/1
  Delay15/1 -> Switch_on7/1
  SampleTime_div_Ly_AXI/1 -> Delay32/1
  Switch_on10/1 -> Delay10/1, MATLAB Function/16(Rs)
  Delay7/1 -> Switch_on7/3
  Delay28/1 -> Switch_on12/3
  Switch_on8/1 -> Delay8/1, MATLAB Function/14(Lq)
  Ld_AXI/1 -> Delay13/1
  Delay6/1 -> Switch_on6/3
  Delay4/1 -> Switch_on4/3
  Switch_on11/1 -> Delay27/1, MATLAB Function/2(SampleTime_div_Lq)
  Delay3/1 -> Switch_on3/3
  Delay14/1 -> Switch_on8/1
  Switch_on2/1 -> Delay2/1, MATLAB Function/1(SampleTime_div_Ld)
  Delay22/1 -> done/1
  Switch_on3/1 -> Delay3/1, Data Type Conversion13/1
  Delay13/1 -> Switch_on9/1
  Delay5/1 -> Switch_on5/3
  SampleTime_div_Ld_AXI/1 -> Delay21/1
  last_applied_optimal_voltages_in/1 -> Delay20/1
  id_measured/1 -> Delay19/1
  iq_measured/1 -> Delay18/1
  ix_measured/1 -> Delay17/1
  iy_measured/1 -> Delay16/1
  omega_m_measured/1 -> Delay34/1
  Delay35/1 -> Detect Rise Positive1/1
  valid_in_ADC/1 -> Delay35/1
  Delay34/1 -> Switch_on14/1
  Delay36/1 -> Switch_on18/1
  Demux/1 -> Data Type Conversion1/1
  Delay37/1 -> Switch_on15/3
  Switch_on15/1 -> MATLAB Function/6(last_applied_optimal_voltage_q), Delay37/1
  Demux/2 -> Data Type Conversion10/1
  Delay38/1 -> Switch_on16/3
  Switch_on16/1 -> MATLAB Function/7(last_applied_optimal_voltage_x), Delay38/1
  Demux/3 -> Data Type Conversion11/1
  Delay39/1 -> Switch_on17/3
  Detect Rise Positive/1 -> Switch_on17/2, Switch_on16/2, Switch_on15/2, Switch_on13/2, Switch_on2/2, Switch_on11/2, Switch_on12/2, Switch_on1/2, Switch_on3/2, Switch_on4/2, Switch_on5/2, Switch_on6/2, Switch_on7/2, Switch_on8/2, Switch_on9/2, Switch_on10/2, Delay22/1  "End_Cycle"
  Switch_on17/1 -> MATLAB Function/8(last_applied_optimal_voltage_y), Delay39/1
  Demux/4 -> Data Type Conversion12/1
  Data Type Conversion1/1 -> Switch_on1/1  "last_applied_optimal_voltage_vector"
  Data Type Conversion10/1 -> Switch_on15/1  "last_applied_optimal_voltage_vector"
  Data Type Conversion11/1 -> Switch_on16/1  "last_applied_optimal_voltage_vector"
  Data Type Conversion12/1 -> Switch_on17/1  "last_applied_optimal_voltage_vector"
  Delay19/1 -> Switch_on3/1
  Delay18/1 -> Switch_on4/1  "last_applied_optimal_voltage_vector"
  Delay17/1 -> Switch_on5/1
  Delay16/1 -> Switch_on6/1
  Data Type Conversion4/1 -> Product/1
  Data Type Conversion/1 -> Delay26/1
  Data Type Conversion7/1 -> Delay25/1
  Data Type Conversion8/1 -> Delay24/1
  Data Type Conversion9/1 -> Delay23/1
  Switch_on18/1 -> Product/2, Delay40/1
  Detect Rise Positive1/1 -> Switch_on18/2, Switch_on14/2  "End_Cycle"
  Delay40/1 -> Switch_on18/3
  Data Type Conversion13/1 -> MATLAB Function/9(id_measured)
  Data Type Conversion14/1 -> MATLAB Function/10(iq_measured)
  Data Type Conversion15/1 -> MATLAB Function/11(ix_measured)
  Data Type Conversion16/1 -> MATLAB Function/12(iy_measured)
  Switch_on7/1 -> MATLAB Function/13(psiPM), Delay7/1
